simulink model "PhysicalLayerModelUSRP"  (R2013b)
settings: Solver=ode3  StartTime=0.0  StopTime=inf  RelTol=1e-3
model workspace (MAT data in the model file):
  CarrierFrequency = Simulink.Parameter
  CarrierFrequency.Value = 2600000
  CarrierFrequency.DataType = 'double'
  SampleTime = Simulink.Parameter
  SampleTime.Value = 1e-06
  SampleTime.DataType = 'double'
  SamplesPerFrame = Simulink.Parameter
  SamplesPerFrame.Value = 264
  SamplesPerFrame.DataType = 'double'
  M_ary = Simulink.Parameter
  M_ary.Value = 16
  M_ary.DataType = 'double'
  DelayParam = Simulink.Parameter
  DelayParam.Value = 2.66
  DelayParam.DataType = 'double'
  SNR = Simulink.Parameter
  SNR.Value = 30
  SNR.DataType = 'double'
  InputSignalPower = Simulink.Parameter
  InputSignalPower.Value = 1
  InputSignalPower.DataType = 'double'
  InterferanceFrequency = Simulink.Parameter
  InterferanceFrequency.Value = 0
  InterferanceFrequency.DataType = 'double'
  SymbolPhaseOffset = Simulink.Parameter
  SymbolPhaseOffset.Value = 0
  SymbolPhaseOffset.DataType = 'double'
  ModulationType = Simulink.Parameter
  ModulationType.Value = 0
  ModulationType.DataType = 'int8'
  SignalPower = Simulink.Parameter
  SignalPower.Value = 1
  SignalPower.DataType = 'double'
undefined symbols (not defined in the file): gcbh, rcfiltgaincompat
libraries: simulink x8, commdigbbndpm3 x4, commfilt2 x4, commdigbbndam3 x4, commsdrhw_v2 x4, dspsrcs4 x2, commtimrec2 x2, dspsigops x2, commsink2 x2
settings Model: BufferReuse=off  Creator=The MathWorks Inc.  LastModifiedBy=Lucas
settings DataIOCC: SignalLoggingSaveFormat=ModelDataLogs  SaveOutput=off  SaveTime=off  SignalLoggingName=logsOut
settings OptimizationCC: OptimizeBlockIOStorage=off  BufferReuse=off  ExpressionFolding=off  ExpressionDepthLimit=2147483647  LocalBlockOutputs=off  InitFltsAndDblsToZero=on
settings DebuggingCC: SaveWithParameterizedLinksMsg=none  MergeDetectMultiDrivingBlocksExec=error  CheckExecutionContextPreStartOutputMsg=on  CheckExecutionContextRuntimeOutputMsg=on  SignalResolutionControl=TryResolveAllWithWarning  SolverPrmCheckMsg=none  InheritedTsInSrcMsg=none  MultiTaskDSMMsg=warning  MultiTaskCondExecSysMsg=none  StateNameClashWarn=warning
settings HardwareCC: ProdHWDeviceType=Specified  TargetLongLongMode=on  TargetIntDivRoundTo=Zero  TargetEndianess=LittleEndian  TargetHWDeviceType=MATLAB Host  ProdEqTarget=off
settings ModelReferenceCC: UpdateModelReferenceTargets=IfOutOfDate
settings RTWCC: GenCodeOnly=on  TemplateMakefile=RTW.MSVCBuild  Description=Create Visual C/C++ Solution File for Simulink Coder  ProcessScript=grt_make_rtw_hook  IncludeERTFirstTime=on  CheckMdlBeforeBuild=Error
settings CodeAppCC: ForceParamTrailComments=on  MangleLength=5  MATLABSourceComments=on
settings GRTTargetCC: CodeReplacementLibrary=C89/C90 (ANSI)  MultiInstanceERTCode=on  GenerateAllocFcn=on  RTWCAPISignals=on  RTWCAPIParams=on

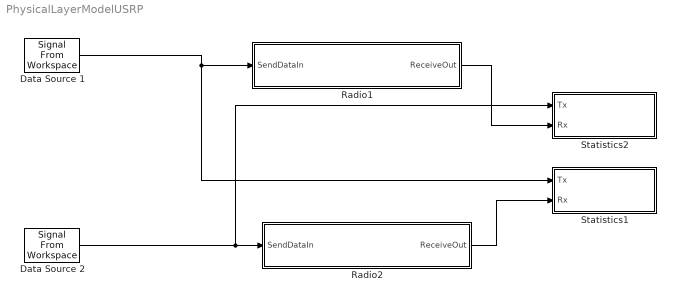
== system PhysicalLayerModelUSRP ==
  Data Source 1 : dspsrcs4/Signal From Workspace  X=data1  Ts=SampleTime  nsamps=SamplesPerFrame  OutputAfterFinalValue=Cyclic repetition  ignoreOrWarnInputAndFrameLengths=on
  Data Source 2 : dspsrcs4/Signal From Workspace  X=data2  Ts=SampleTime  nsamps=SamplesPerFrame  OutputAfterFinalValue=Cyclic repetition  ignoreOrWarnInputAndFrameLengths=on
  Radio1 : Subsystem
  Radio2 : Subsystem
  Statistics1 : Subsystem  TreatAsAtomicUnit=on
      settings: RTWFcnNameOpts=Use subsystem name  RTWFileNameOpts=Use function name
  Statistics2 : Subsystem  TreatAsAtomicUnit=on
      settings: RTWFcnNameOpts=Use subsystem name  RTWFileNameOpts=Use function name
  wires:
  Data Source 1/1 -> Statistics1/1(Tx), Radio1/1(SendDataIn)
  Data Source 2/1 -> Radio2/1(SendDataIn), Statistics2/1(Tx)
  Radio2/1(ReceiveOut) -> Statistics1/2(Rx)
  Radio1/1(ReceiveOut) -> Statistics2/2(Rx)

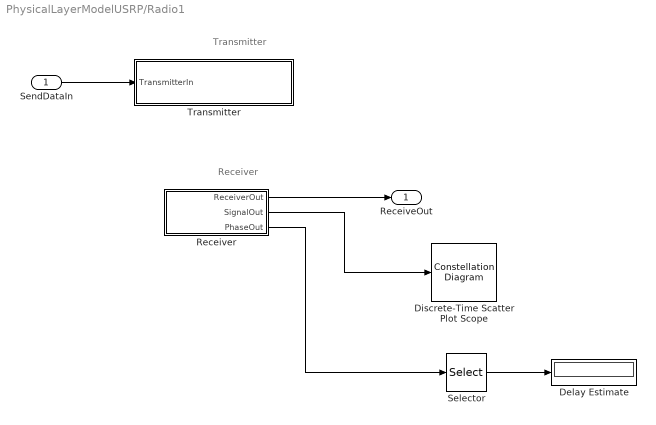
== system PhysicalLayerModelUSRP/Radio1 ==
  note: Transmitter
  note: Receiver
  SendDataIn : Inport
  Delay Estimate : Display
  Discrete-Time Scatter Plot Scope : ConstellationDiagram  Tag=ScatterPlot
      settings: CopyFcn=scopeextensions.ScopeBlock.onCoreBlockCopy(gcbh);  DeleteFcn=scopeextensions.ScopeBlock.callback(gcbh, 'onBlockDelete');  PreSaveFcn=scopeextensions.ScopeBlock.callback(gcbh, 'onModelSave');  NameChangeFcn=scopeextensions.ScopeBlock.callback(gcbh, 'onBlockRename');  DestroyFcn=scopeextensions.ScopeBlock.onBlockDestroy(gcbh)  CloseFcn=scopeextensions.ScopeBlock.callback(gcbh, 'onBlockClose');  PreDeleteFcn=scopeextensions.ScopeBlock.callback(gcbh, 'onBlockPreDelete');
  Receiver : Subsystem  TreatAsAtomicUnit=on
      settings: RTWFcnNameOpts=Use subsystem name  RTWFileNameOpts=Use function name
  Selector : Selector  InputPortWidth=SamplesPerFrame  IndexOptions=Index vector (dialog)  Indices=1  OutputSizes=1
  Transmitter : Subsystem  TreatAsAtomicUnit=on
      settings: RTWFcnNameOpts=Use subsystem name  RTWFileNameOpts=Use function name
  ReceiveOut : Outport
  wires:
  SendDataIn/1 -> Transmitter/1(TransmitterIn)
  Receiver/1(ReceiverOut) -> ReceiveOut/1
  Selector/1 -> Delay Estimate/1
  Receiver/2(SignalOut) -> Discrete-Time Scatter Plot Scope/1
  Receiver/3(PhaseOut) -> Selector/1

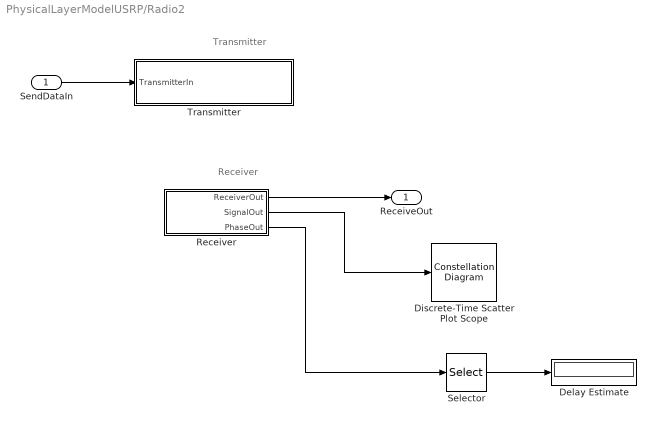
== system PhysicalLayerModelUSRP/Radio2 ==
  note: Transmitter
  note: Receiver
  SendDataIn : Inport
  Delay Estimate : Display
  Discrete-Time Scatter Plot Scope : ConstellationDiagram  Tag=ScatterPlot
      settings: CopyFcn=scopeextensions.ScopeBlock.onCoreBlockCopy(gcbh);  DeleteFcn=scopeextensions.ScopeBlock.callback(gcbh, 'onBlockDelete');  PreSaveFcn=scopeextensions.ScopeBlock.callback(gcbh, 'onModelSave');  NameChangeFcn=scopeextensions.ScopeBlock.callback(gcbh, 'onBlockRename');  DestroyFcn=scopeextensions.ScopeBlock.onBlockDestroy(gcbh)  CloseFcn=scopeextensions.ScopeBlock.callback(gcbh, 'onBlockClose');  PreDeleteFcn=scopeextensions.ScopeBlock.callback(gcbh, 'onBlockPreDelete');
  Receiver : Subsystem  TreatAsAtomicUnit=on
      settings: RTWFcnNameOpts=Use subsystem name  RTWFileNameOpts=Use function name
  Selector : Selector  InputPortWidth=SamplesPerFrame  IndexOptions=Index vector (dialog)  Indices=1  OutputSizes=1
  Transmitter : Subsystem  TreatAsAtomicUnit=on
      settings: RTWFcnNameOpts=Use subsystem name  RTWFileNameOpts=Use function name
  ReceiveOut : Outport
  wires:
  SendDataIn/1 -> Transmitter/1(TransmitterIn)
  Receiver/1(ReceiverOut) -> ReceiveOut/1
  Selector/1 -> Delay Estimate/1
  Receiver/2(SignalOut) -> Discrete-Time Scatter Plot Scope/1
  Receiver/3(PhaseOut) -> Selector/1

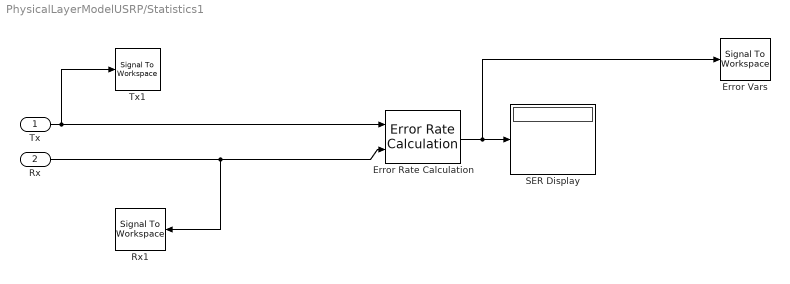
== system PhysicalLayerModelUSRP/Statistics1 ==
  Tx : Inport
  Rx : Inport  Port=2
  Error Rate Calculation : commsink2/Error Rate Calculation  N=8  st_delay=0  cp_mode=Entire frame  subframe=[]  PMode=Port  WsName=ErrorVec  RsMode2=off  stop=off  numErr=100  maxBits=1e6
  Error Vars : SignalToWorkspace  VariableName=ErrorVars1
      settings: CopyFcn=dspblkcopystw(gcbh);
  Rx1 : SignalToWorkspace  VariableName=Rx1
      settings: CopyFcn=dspblkcopystw(gcbh);
  SER Display : Display
  Tx1 : SignalToWorkspace  VariableName=Tx1
      settings: CopyFcn=dspblkcopystw(gcbh);
  wires:
  Error Rate Calculation/1 -> Error Vars/1, SER Display/1
  Tx/1 -> Tx1/1, Error Rate Calculation/1
  Rx/1 -> Rx1/1, Error Rate Calculation/2

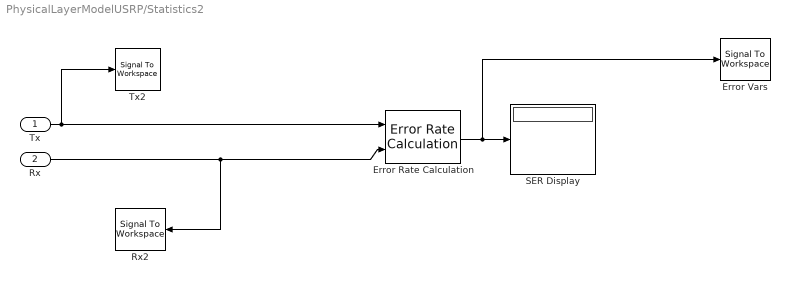
== system PhysicalLayerModelUSRP/Statistics2 ==
  Tx : Inport
  Rx : Inport  Port=2
  Error Rate Calculation : commsink2/Error Rate Calculation  N=8  st_delay=0  cp_mode=Entire frame  subframe=[]  PMode=Port  WsName=ErrorVec  RsMode2=off  stop=off  numErr=100  maxBits=1e6
  Error Vars : SignalToWorkspace  VariableName=ErrorVars2
      settings: CopyFcn=dspblkcopystw(gcbh);
  Rx2 : SignalToWorkspace  VariableName=Rx2
      settings: CopyFcn=dspblkcopystw(gcbh);
  SER Display : Display
  Tx2 : SignalToWorkspace  VariableName=Tx2
      settings: CopyFcn=dspblkcopystw(gcbh);
  wires:
  Error Rate Calculation/1 -> Error Vars/1, SER Display/1
  Tx/1 -> Tx2/1, Error Rate Calculation/1
  Rx/1 -> Rx2/1, Error Rate Calculation/2

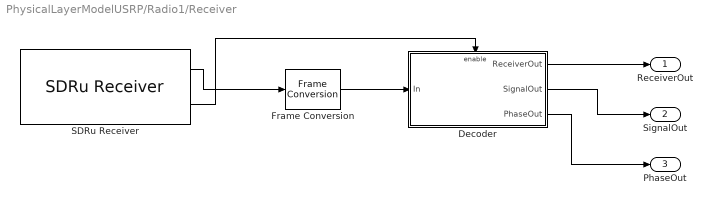
== system PhysicalLayerModelUSRP/Radio1/Receiver ==
  Decoder : Subsystem  TreatAsAtomicUnit=on
  Frame Conversion : FrameConversion
  SDRu Receiver : commsdrhw_v2/SDRu Receiver  rxtx=rx  USRP2_IP='192.168.10.2'  centerFrequency=CarrierFrequency  centerFrequencySrc=Dialog  loOffset=0  loOffsetSrc=Dialog  gain=SignalPower  gainSrc=Dialog  decimInterp=1  decimInterpSrc=Dialog  USRP2_IP_NUM=[49 57 50 46 49 54 56 46 49 48 46 50]  frameLength=SamplesPerFrame*8  outputDatatype=double  overrunUnderrunPort=off  sampleTime=SampleTime/8  HOST_DATA_PORT=0  HOST_CONTROL_PORT=0  USRP2_DATA_PORT=0  USRP2_CONTROL_PORT=0  bufferMode=Continuous streaming  EnableBurstMode=off  NumFramesInBurst=100
  ReceiverOut : Outport
  SignalOut : Outport  Port=2
  PhaseOut : Outport  Port=3
  wires:
  Decoder/1(ReceiverOut) -> ReceiverOut/1
  Decoder/2(SignalOut) -> SignalOut/1
  Decoder/3(PhaseOut) -> PhaseOut/1
  SDRu Receiver/2 -> Decoder/Enable
  Frame Conversion/1 -> Decoder/1(In)
  SDRu Receiver/1 -> Frame Conversion/1

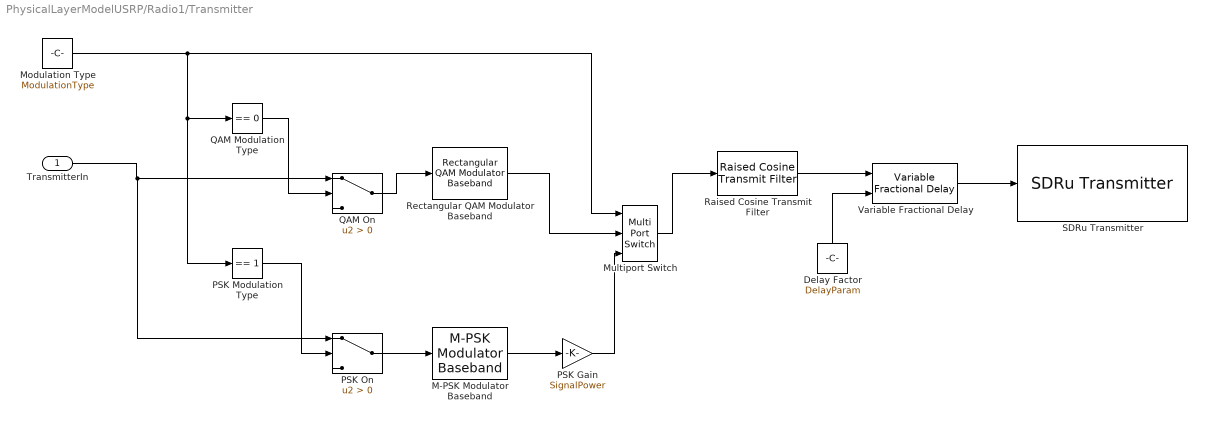
== system PhysicalLayerModelUSRP/Radio1/Transmitter ==
  TransmitterIn : Inport
  Delay Factor : Constant  Value=DelayParam
  M-PSK Modulator Baseband : commdigbbndpm3/M-PSK Modulator Baseband  M=M_ary  InType=Integer  Enc=Gray  Mapping=[0:7]  Ph=pi/M_ary  outDtype=double  outWordLen=16  outUDDataType=sfix(16)  outFracLenMode=Best precision  outFracLen=15
  Modulation Type : Constant  Value=ModulationType
  Multiport Switch : MultiPortSwitch  DataPortOrder=Zero-based contiguous  Inputs=2
  PSK Gain : Gain  Gain=SignalPower
  PSK Modulation Type : simulink/Logic and Bit Operations/Compare To Constant  relop===  const=1  OutDataTypeStr=uint8
  PSK On : Switch  Criteria=u2 > Threshold
  QAM Modulation Type : simulink/Logic and Bit Operations/Compare To Constant  relop===  const=0  OutDataTypeStr=uint8
  QAM On : Switch  Criteria=u2 > Threshold
  Raised Cosine Transmit Filter : commfilt2/Raised Cosine Transmit Filter  filtType=Square root  filtSpan=2*(4)  currentFiltSpan=2*(4)  D=(2*(4))/2  R=0.2  sampMode=Mute  saveAsFlag=0  N=8  framing=Enforce single-rate processing  InputProcessing=Columns as channels (frame based)  checkGain=Normalized  filterGain=rcfiltgaincompat(gcbh)  checkCoeff=off  variableName=rcTxFilt  launchFVT=off  roundingMode=Floor  overflowMode=off
  Rectangular QAM Modulator Baseband : commdigbbndam3/Rectangular QAM Modulator Baseband  M=M_ary  InType=Integer  Enc=Binary  Mapping=[0:15]  PowType=Min. distance between symbols  MinDist=SignalPower  AvgPow=1  PeakPow=1  Ph=SymbolPhaseOffset  outDtype=double  outWordLen=16  outUDDataType=sfix(16)  outFracLenMode=Best precision  outFracLen=15
  SDRu Transmitter : commsdrhw_v2/SDRu Transmitter  rxtx=tx  USRP2_IP='192.168.10.2'  centerFrequency=CarrierFrequency  centerFrequencySrc=Dialog  loOffset=0  loOffsetSrc=Dialog  gain=SignalPower  gainSrc=Dialog  decimInterp=1e8*SampleTime  decimInterpSrc=Dialog  USRP2_IP_NUM=[49 57 50 46 49 54 56 46 49 48 46 50]  frameLength=362  outputDatatype=int16  overrunUnderrunPort=off  sampleTime=1  dboardInfo=|  HOST_DATA_PORT=30000  HOST_CONTROL_PORT=30001  USRP2_DATA_PORT=32769  USRP2_CONTROL_PORT=32768  bufferMode=Continuous streaming  EnableBurstMode=off  NumFramesInBurst=100
      | dbid: 0
      |           dbName: 'no db found'
      |          freqMin: 0
      |          freqMax: 0
      |          gainMin: 0
      |          gainMax: 0
      |     gainStepSize: 0
  Variable Fractional Delay : dspsigops/Variable Fractional Delay  mode=OBSOLETE  modeActive=Linear  dmax=4  InputProcessing=Columns as channels (frame based)  L=4  FarrowL=4  R=10  alpha=1  ic=0  fallbackFIR=Clip to the minimum value necessary for centered kernel  fallbackFarrow=Clip to the minimum value necessary for centered kernel  noDFT=off  roundingMode=Zero  overflowMode=off
  wires:
  Delay Factor/1 -> Variable Fractional Delay/2
  Raised Cosine Transmit Filter/1 -> Variable Fractional Delay/1
  Variable Fractional Delay/1 -> SDRu Transmitter/1
  Multiport Switch/1 -> Raised Cosine Transmit Filter/1
  Rectangular QAM Modulator Baseband/1 -> Multiport Switch/2
  Modulation Type/1 -> PSK Modulation Type/1, QAM Modulation Type/1, Multiport Switch/1
  TransmitterIn/1 -> PSK On/1, QAM On/1
  QAM On/1 -> Rectangular QAM Modulator Baseband/1
  PSK On/1 -> M-PSK Modulator Baseband/1
  QAM Modulation Type/1 -> QAM On/2
  PSK Modulation Type/1 -> PSK On/2
  M-PSK Modulator Baseband/1 -> PSK Gain/1
  PSK Gain/1 -> Multiport Switch/3

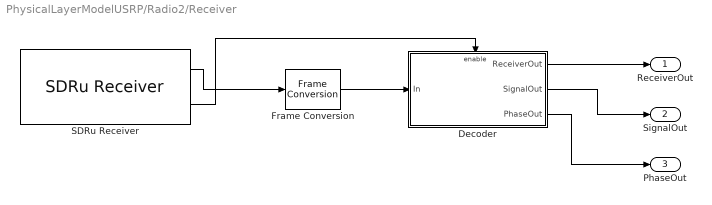
== system PhysicalLayerModelUSRP/Radio2/Receiver ==
  Decoder : Subsystem  TreatAsAtomicUnit=on
  Frame Conversion : FrameConversion
  SDRu Receiver : commsdrhw_v2/SDRu Receiver  rxtx=rx  USRP2_IP='192.168.10.2'  centerFrequency=CarrierFrequency  centerFrequencySrc=Dialog  loOffset=0  loOffsetSrc=Dialog  gain=SignalPower  gainSrc=Dialog  decimInterp=1  decimInterpSrc=Dialog  USRP2_IP_NUM=[49 57 50 46 49 54 56 46 49 48 46 50]  frameLength=SamplesPerFrame*8  outputDatatype=double  overrunUnderrunPort=off  sampleTime=SampleTime/8  HOST_DATA_PORT=0  HOST_CONTROL_PORT=0  USRP2_DATA_PORT=0  USRP2_CONTROL_PORT=0  bufferMode=Continuous streaming  EnableBurstMode=off  NumFramesInBurst=100
  ReceiverOut : Outport
  SignalOut : Outport  Port=2
  PhaseOut : Outport  Port=3
  wires:
  Decoder/1(ReceiverOut) -> ReceiverOut/1
  Decoder/2(SignalOut) -> SignalOut/1
  Decoder/3(PhaseOut) -> PhaseOut/1
  SDRu Receiver/2 -> Decoder/Enable
  Frame Conversion/1 -> Decoder/1(In)
  SDRu Receiver/1 -> Frame Conversion/1

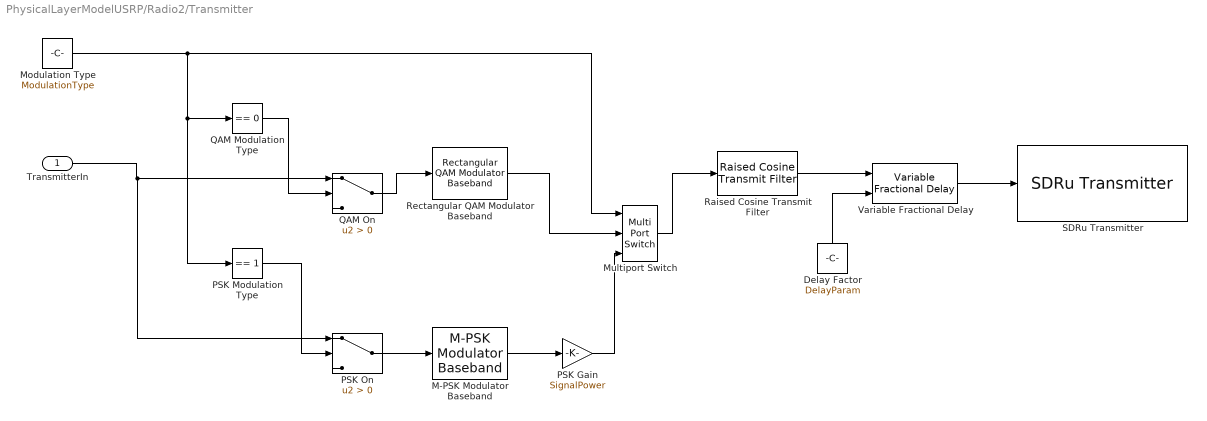
== system PhysicalLayerModelUSRP/Radio2/Transmitter ==
  TransmitterIn : Inport
  Delay Factor : Constant  Value=DelayParam
  M-PSK Modulator Baseband : commdigbbndpm3/M-PSK Modulator Baseband  M=M_ary  InType=Integer  Enc=Gray  Mapping=[0:7]  Ph=pi/M_ary  outDtype=double  outWordLen=16  outUDDataType=sfix(16)  outFracLenMode=Best precision  outFracLen=15
  Modulation Type : Constant  Value=ModulationType
  Multiport Switch : MultiPortSwitch  DataPortOrder=Zero-based contiguous  Inputs=2
  PSK Gain : Gain  Gain=SignalPower
  PSK Modulation Type : simulink/Logic and Bit Operations/Compare To Constant  relop===  const=1  OutDataTypeStr=uint8
  PSK On : Switch  Criteria=u2 > Threshold
  QAM Modulation Type : simulink/Logic and Bit Operations/Compare To Constant  relop===  const=0  OutDataTypeStr=uint8
  QAM On : Switch  Criteria=u2 > Threshold
  Raised Cosine Transmit Filter : commfilt2/Raised Cosine Transmit Filter  filtType=Square root  filtSpan=2*(4)  currentFiltSpan=2*(4)  D=(2*(4))/2  R=0.2  sampMode=Mute  saveAsFlag=0  N=8  framing=Enforce single-rate processing  InputProcessing=Columns as channels (frame based)  checkGain=Normalized  filterGain=rcfiltgaincompat(gcbh)  checkCoeff=off  variableName=rcTxFilt  launchFVT=off  roundingMode=Floor  overflowMode=off
  Rectangular QAM Modulator Baseband : commdigbbndam3/Rectangular QAM Modulator Baseband  M=M_ary  InType=Integer  Enc=Binary  Mapping=[0:15]  PowType=Min. distance between symbols  MinDist=SignalPower  AvgPow=1  PeakPow=1  Ph=SymbolPhaseOffset  outDtype=double  outWordLen=16  outUDDataType=sfix(16)  outFracLenMode=Best precision  outFracLen=15
  SDRu Transmitter : commsdrhw_v2/SDRu Transmitter  rxtx=tx  USRP2_IP='192.168.10.2'  centerFrequency=CarrierFrequency  centerFrequencySrc=Dialog  loOffset=0  loOffsetSrc=Dialog  gain=SignalPower  gainSrc=Dialog  decimInterp=1e8*SampleTime  decimInterpSrc=Dialog  USRP2_IP_NUM=[49 57 50 46 49 54 56 46 49 48 46 50]  frameLength=362  outputDatatype=int16  overrunUnderrunPort=off  sampleTime=1  dboardInfo=|  HOST_DATA_PORT=30000  HOST_CONTROL_PORT=30001  USRP2_DATA_PORT=32769  USRP2_CONTROL_PORT=32768  bufferMode=Continuous streaming  EnableBurstMode=off  NumFramesInBurst=100
      | dbid: 0
      |           dbName: 'no db found'
      |          freqMin: 0
      |          freqMax: 0
      |          gainMin: 0
      |          gainMax: 0
      |     gainStepSize: 0
  Variable Fractional Delay : dspsigops/Variable Fractional Delay  mode=OBSOLETE  modeActive=Linear  dmax=4  InputProcessing=Columns as channels (frame based)  L=4  FarrowL=4  R=10  alpha=1  ic=0  fallbackFIR=Clip to the minimum value necessary for centered kernel  fallbackFarrow=Clip to the minimum value necessary for centered kernel  noDFT=off  roundingMode=Zero  overflowMode=off
  wires:
  Delay Factor/1 -> Variable Fractional Delay/2
  Raised Cosine Transmit Filter/1 -> Variable Fractional Delay/1
  Variable Fractional Delay/1 -> SDRu Transmitter/1
  Multiport Switch/1 -> Raised Cosine Transmit Filter/1
  Rectangular QAM Modulator Baseband/1 -> Multiport Switch/2
  Modulation Type/1 -> PSK Modulation Type/1, QAM Modulation Type/1, Multiport Switch/1
  TransmitterIn/1 -> PSK On/1, QAM On/1
  QAM On/1 -> Rectangular QAM Modulator Baseband/1
  PSK On/1 -> M-PSK Modulator Baseband/1
  QAM Modulation Type/1 -> QAM On/2
  PSK Modulation Type/1 -> PSK On/2
  M-PSK Modulator Baseband/1 -> PSK Gain/1
  PSK Gain/1 -> Multiport Switch/3

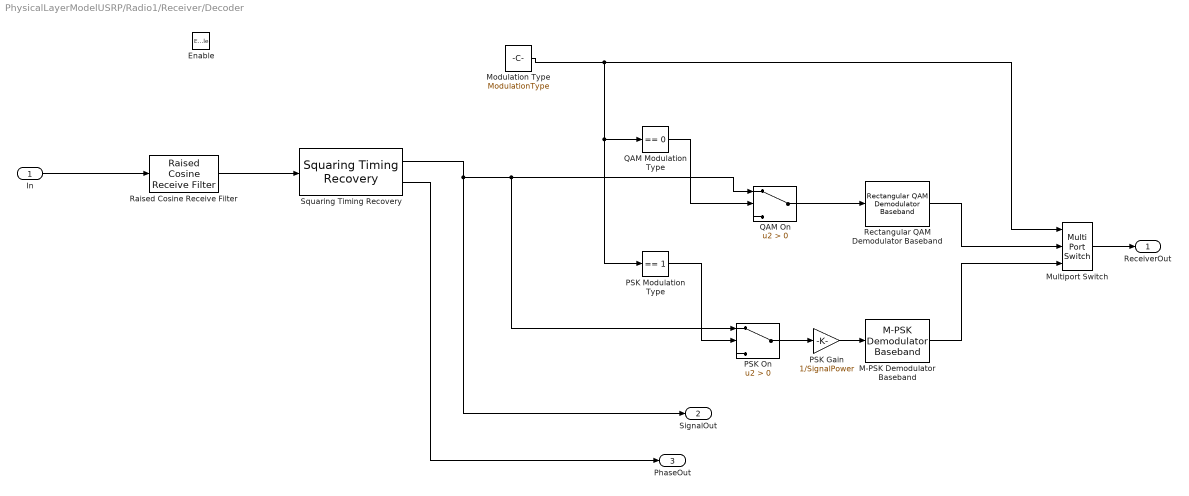
== system PhysicalLayerModelUSRP/Radio1/Receiver/Decoder ==
  In : Inport
  Enable : EnablePort
  M-PSK Demodulator Baseband : commdigbbndpm3/M-PSK Demodulator Baseband  M=M_ary  Ph=pi/M_ary  Dec=Gray  Mapping=[0:7]  OutType=Integer  DecType=Hard decision  VarSource=Dialog  Variance=1  outDtype1=Inherit via internal rule  outDtype2=uint8  derotateFactorWordLen=16
  Modulation Type : Constant  Value=ModulationType
  Multiport Switch : MultiPortSwitch  DataPortOrder=Zero-based contiguous  Inputs=2
  PSK Gain : Gain  Gain=1/SignalPower
  PSK Modulation Type : simulink/Logic and Bit Operations/Compare To Constant  relop===  const=1  OutDataTypeStr=uint8
  PSK On : Switch  Criteria=u2 > Threshold
  QAM Modulation Type : simulink/Logic and Bit Operations/Compare To Constant  relop===  const=0  OutDataTypeStr=uint8
  QAM On : Switch  Criteria=u2 > Threshold
  Raised Cosine Receive Filter : commfilt2/Raised Cosine Receive Filter  filtType=Square root  N=8  filtSpan=2*(4)  currentFiltSpan=2*(4)  D=4  R=0.2  sampMode=Mute  saveAsFlag=0  rateMode=Downsampling  downFactor=1  downOffset=0  framing=Maintain input frame rate  InputProcessing=Columns as channels (frame based)  checkGain=Normalized  filterGain=rcfiltgaincompat(gcbh)  checkCoeff=off  variableName=rcRxFilt  launchFVT=off  roundingMode=Floor  overflowMode=off
  Rectangular QAM Demodulator Baseband : commdigbbndam3/Rectangular QAM Demodulator Baseband  M=M_ary  PowType=Min. distance between symbols  MinDist=SignalPower  AvgPow=1  PeakPow=1  Ph=SymbolPhaseOffset  Dec=Binary  Mapping=[0:15]  OutType=Integer  DecType=Hard decision  VarSource=Dialog  Variance=1  outDtype1=double  outDtype2=uint8  derotateFactorWordLen=16  denormFactorWordLen=16  prodOutWordLen=32  prodOutRoundingMode=Floor  prodOutOverflowMode=Wrap  sumWordLen=32
  Squaring Timing Recovery : commtimrec2/Squaring Timing Recovery  numSymb=SamplesPerFrame  sampPerSymb=8
  ReceiverOut : Outport
  SignalOut : Outport  Port=2
  PhaseOut : Outport  Port=3
  wires:
  Squaring Timing Recovery/2 -> PhaseOut/1
  Raised Cosine Receive Filter/1 -> Squaring Timing Recovery/1
  Rectangular QAM Demodulator Baseband/1 -> Multiport Switch/2
  M-PSK Demodulator Baseband/1 -> Multiport Switch/3
  Multiport Switch/1 -> ReceiverOut/1
  QAM On/1 -> Rectangular QAM Demodulator Baseband/1
  Squaring Timing Recovery/1 -> PSK On/1, QAM On/1, SignalOut/1
  Modulation Type/1 -> PSK Modulation Type/1, QAM Modulation Type/1, Multiport Switch/1
  QAM Modulation Type/1 -> QAM On/2
  PSK Modulation Type/1 -> PSK On/2
  PSK On/1 -> PSK Gain/1
  PSK Gain/1 -> M-PSK Demodulator Baseband/1
  In/1 -> Raised Cosine Receive Filter/1

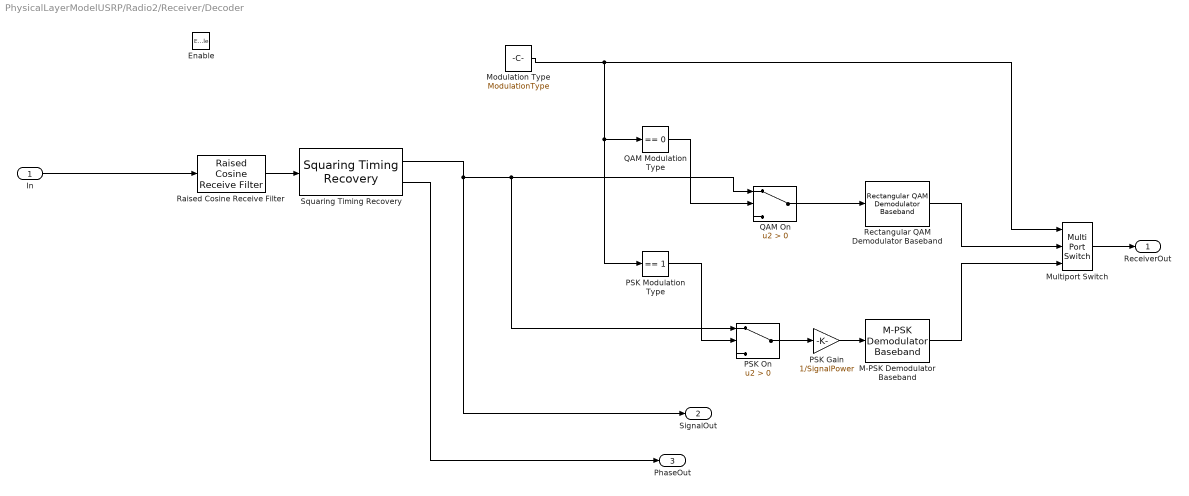
== system PhysicalLayerModelUSRP/Radio2/Receiver/Decoder ==
  In : Inport
  Enable : EnablePort
  M-PSK Demodulator Baseband : commdigbbndpm3/M-PSK Demodulator Baseband  M=M_ary  Ph=pi/M_ary  Dec=Gray  Mapping=[0:7]  OutType=Integer  DecType=Hard decision  VarSource=Dialog  Variance=1  outDtype1=Inherit via internal rule  outDtype2=uint8  derotateFactorWordLen=16
  Modulation Type : Constant  Value=ModulationType
  Multiport Switch : MultiPortSwitch  DataPortOrder=Zero-based contiguous  Inputs=2
  PSK Gain : Gain  Gain=1/SignalPower
  PSK Modulation Type : simulink/Logic and Bit Operations/Compare To Constant  relop===  const=1  OutDataTypeStr=uint8
  PSK On : Switch  Criteria=u2 > Threshold
  QAM Modulation Type : simulink/Logic and Bit Operations/Compare To Constant  relop===  const=0  OutDataTypeStr=uint8
  QAM On : Switch  Criteria=u2 > Threshold
  Raised Cosine Receive Filter : commfilt2/Raised Cosine Receive Filter  filtType=Square root  N=8  filtSpan=2*(4)  currentFiltSpan=2*(4)  D=4  R=0.2  sampMode=Mute  saveAsFlag=0  rateMode=Downsampling  downFactor=1  downOffset=0  framing=Maintain input frame rate  InputProcessing=Columns as channels (frame based)  checkGain=Normalized  filterGain=rcfiltgaincompat(gcbh)  checkCoeff=off  variableName=rcRxFilt  launchFVT=off  roundingMode=Floor  overflowMode=off
  Rectangular QAM Demodulator Baseband : commdigbbndam3/Rectangular QAM Demodulator Baseband  M=M_ary  PowType=Min. distance between symbols  MinDist=SignalPower  AvgPow=1  PeakPow=1  Ph=SymbolPhaseOffset  Dec=Binary  Mapping=[0:15]  OutType=Integer  DecType=Hard decision  VarSource=Dialog  Variance=1  outDtype1=double  outDtype2=uint8  derotateFactorWordLen=16  denormFactorWordLen=16  prodOutWordLen=32  prodOutRoundingMode=Floor  prodOutOverflowMode=Wrap  sumWordLen=32
  Squaring Timing Recovery : commtimrec2/Squaring Timing Recovery  numSymb=SamplesPerFrame  sampPerSymb=8
  ReceiverOut : Outport
  SignalOut : Outport  Port=2
  PhaseOut : Outport  Port=3
  wires:
  Squaring Timing Recovery/2 -> PhaseOut/1
  Raised Cosine Receive Filter/1 -> Squaring Timing Recovery/1
  Rectangular QAM Demodulator Baseband/1 -> Multiport Switch/2
  M-PSK Demodulator Baseband/1 -> Multiport Switch/3
  Multiport Switch/1 -> ReceiverOut/1
  QAM On/1 -> Rectangular QAM Demodulator Baseband/1
  Squaring Timing Recovery/1 -> PSK On/1, QAM On/1, SignalOut/1
  Modulation Type/1 -> PSK Modulation Type/1, QAM Modulation Type/1, Multiport Switch/1
  QAM Modulation Type/1 -> QAM On/2
  PSK Modulation Type/1 -> PSK On/2
  PSK On/1 -> PSK Gain/1
  PSK Gain/1 -> M-PSK Demodulator Baseband/1
  In/1 -> Raised Cosine Receive Filter/1
